simulink model "Verifica_HINF"  (R2025b)
settings: Solver=VariableStepAuto  StartTime=0.0  StopTime=1e3  RelTol=1e-3
libraries: cstblocks x2
settings Model: Creator=salvo  LastModifiedBy=salvo

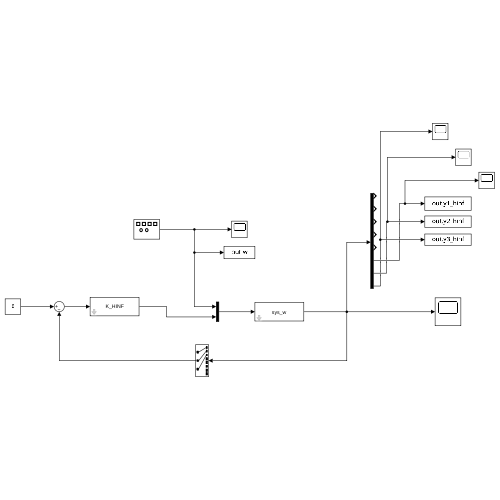
[thumbnail: Simulink's stored preview of the top-level diagram]
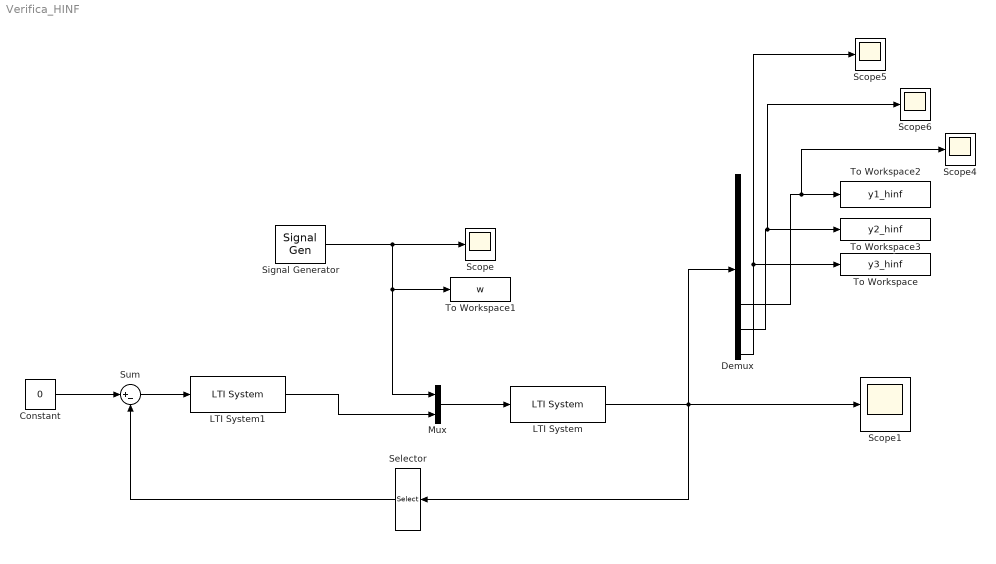
== system Verifica_HINF ==
  Constant : Constant  Value=0
  Demux : Demux  Outputs=8
  LTI System : cstblocks/LTI System  sys=sys_w  IC=h0  PadeOrder=0
  LTI System1 : cstblocks/LTI System  sys=K_HINF  IC=[]  PadeOrder=0
  Mux : Mux  Inputs=2
  Scope{,1,4..6} (5 alike) : Scope
      Scope settings: ActiveDisplayYMinimum=-2.3885392133233507  ActiveDisplayYMaximum=3.068633022970733
      Scope1 settings: ActiveDisplayYMinimum=-16.949223505413645  ActiveDisplayYMaximum=15.69800608849086
      Scope4 settings: ActiveDisplayYMinimum=-1.7261594622847767  ActiveDisplayYMaximum=3.5808651957856084  DataLoggingVariableName=ScopeData4
      Scope5 settings: ActiveDisplayYMinimum=-1.4029213999231773  ActiveDisplayYMaximum=2.9106332592949298  DataLoggingVariableName=ScopeData5
      Scope6 settings: ActiveDisplayYMinimum=-1.8616829801263051  ActiveDisplayYMaximum=2.0355439883479618  DataLoggingVariableName=ScopeData6
  Selector : Selector  InputPortWidth=8  IndexOptions=Index vector (dialog)  Indices=[1 2 3]  OutputSizes=1
  Signal Generator : SignalGenerator  Amplitude=5  Units=rad/sec
  Sum : Sum  Inputs=|+-
  To Workspace : ToWorkspace  VariableName=y3_hinf  SaveFormat=Timeseries  SampleTime=-1
  To Workspace1 : ToWorkspace  VariableName=w  SaveFormat=Timeseries  SampleTime=-1
  To Workspace2 : ToWorkspace  VariableName=y1_hinf  SaveFormat=Timeseries  SampleTime=-1
  To Workspace3 : ToWorkspace  VariableName=y2_hinf  SaveFormat=Timeseries  SampleTime=-1
  wires:
  Mux/1 -> LTI System/1
  LTI System/1 -> Selector/1, Demux/1, Scope1/1
  Constant/1 -> Sum/1
  Sum/1 -> LTI System1/1
  Signal Generator/1 -> Mux/1, To Workspace1/1, Scope/1
  Selector/1 -> Sum/2
  Demux/6 -> Scope4/1, To Workspace2/1
  Demux/7 -> Scope6/1, To Workspace3/1
  Demux/8 -> Scope5/1, To Workspace/1
  LTI System1/1 -> Mux/2
